simulink model "Regler_und_reale_Strecke"  (Simulink 7.0)
settings: Solver=FixedStepDiscrete  SolverMode=SingleTasking  StartTime=0.0  StopTime=20  FixedStep=0.001  RelTol=1e-3
undefined symbols (not defined in the file): National_Instruments, PCI
libraries: rtwinlib x2
settings Model: Creator=Admin  LastModifiedBy=Student  SimulationMode=external  ExtModeTrigDuration=1000000
settings OptimizationCC: InlineInvariantSignals=on
settings DebuggingCC: SaveWithParameterizedLinksMsg=none  SignalResolutionControl=TryResolveAllWithWarning  MultiTaskDSMMsg=warning  MultiTaskCondExecSysMsg=none  StrictBusMsg=None
settings RTWCC: SystemTargetFile=rtwin.tlc  TemplateMakefile=rtwin.tmf  Description=Real-Time Windows Target  ProcessScript=rtwin_make_rtw_hook  IncludeERTFirstTime=on
settings RTWinTargetCC: TargetFcnLib=ansi_tfl_tmw.mat  GenFloatMathFcnCalls=ANSI_C  ModelReferenceCompliant=off  CompOptLevelCompliant=off  PortableWordSizes=off  CCOptimize=on  RebuildAll=on  ExtModeStaticAlloc=on

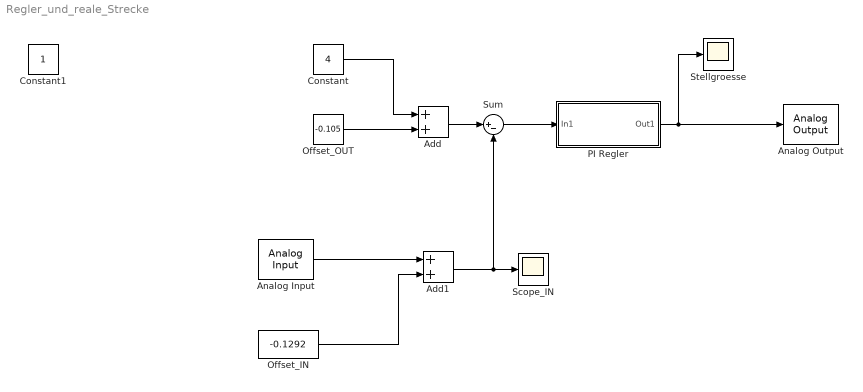
== system Regler_und_reale_Strecke ==
  Add : Sum  OutDataType=sfix(16)  OutScaling=2^-10
  Add1 : Sum  OutDataType=sfix(16)  OutScaling=2^-10
  Analog Input : rtwinlib/Analog Input  SampleTime=0.001  DrvName=National_Instruments/PCI-6025E  DrvAddress=4294967295  DrvOptions=[0 1 0 0 0 0]  Channels=1  RangeMode=1  VoltRange=1  DataType=1
      settings: AttributesFormatString=National Instruments\nPCI-6025E [auto]
  Analog Output : rtwinlib/Analog Output  SampleTime=0.001  DrvName=National_Instruments/PCI-6025E  DrvAddress=4294967295  DrvOptions=[0 1 0 0 0 0]  Channels=1  RangeMode=1  VoltRange=1  InitialValue=0  FinalValue=0
      settings: AttributesFormatString=National Instruments\nPCI-6025E [auto]
  Constant : Constant  Value=4  OutDataType=sfix(16)  OutScaling=2^0
  Offset_IN : Constant  Value=-0.1292  OutDataType=sfix(16)  OutScaling=2^0
  Offset_OUT : Constant  Value=-0.105  OutDataType=sfix(16)  OutScaling=2^0
  PI Regler : Subsystem
  Scope_IN : Scope
      settings: TimeRange=1  YMin=3.5  YMax=4.5  SaveName=ScopeIn_sprungant  DataFormat=Array
  Stellgroesse : Scope
      settings: TimeRange=1  YMin=2.5  YMax=3.5  SaveName=ScopeOut1  DataFormat=Array
  Sum : Sum  Inputs=|+-  OutDataType=sfix(16)  OutScaling=2^0
  Constant1 : Constant  IOType=siggen  OutDataType=sfix(16)  OutScaling=2^0
  wires:
  Analog Input/1 -> Add1/1
  Offset_OUT/1 -> Add/2
  Offset_IN/1 -> Add1/2
  Constant/1 -> Add/1
  PI Regler/1(Out1) -> Analog Output/1, Stellgroesse/1
  Add/1 -> Sum/1
  Sum/1 -> PI Regler/1(In1)
  Add1/1 -> Sum/2, Scope_IN/1

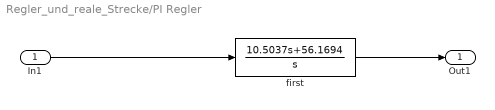
== system Regler_und_reale_Strecke/PI Regler ==
  In1 : Inport  OutDataType=sfix(16)  OutScaling=2^0
  first : TransferFcn  Numerator=[10.5037 56.1694]  Denominator=[1 0]
  Out1 : Outport  OutDataType=sfix(16)  OutScaling=2^0
  wires:
  In1/1 -> first/1
  first/1 -> Out1/1
